simulink library "quat_err_lib"  (R2018b)
settings: Solver=VariableStepAuto  StartTime=0.0  StopTime=10.0  RelTol=1e-3
libraries: aerolibutil x2
settings Model: Creator=Taylor  LastModifiedBy=Taylor

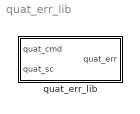
== system quat_err_lib ==
  quat_err_lib : Subsystem  TreatAsAtomicUnit=on
      settings: RTWFcnNameOpts=Use subsystem name  RTWFileNameOpts=Use subsystem name

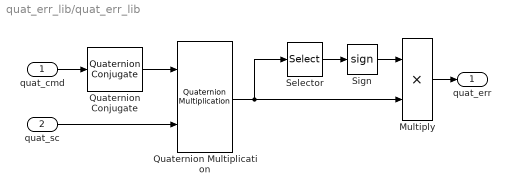
== system quat_err_lib/quat_err_lib ==
  quat_cmd : Inport
  quat_sc : Inport  Port=2
  Multiply : Product
  Quaternion Conjugate : aerolibutil/Quaternion Conjugate
      settings: SourceProductName=Aerospace Blockset  SourceProductBaseCode=AE
  Quaternion Multiplication : aerolibutil/Quaternion Multiplication
  Selector : Selector  InputPortWidth=4  IndexOptions=Index vector (dialog)  Indices=[1]  OutputSizes=1
  Sign : Signum
  quat_err : Outport
  wires:
  Quaternion Conjugate/1 -> Quaternion Multiplication/1
  quat_cmd/1 -> Quaternion Conjugate/1
  Sign/1 -> Multiply/1
  Quaternion Multiplication/1 -> Multiply/2, Selector/1
  quat_sc/1 -> Quaternion Multiplication/2
  Multiply/1 -> quat_err/1
  Selector/1 -> Sign/1
